simulink model "Sim_unicycle"  (R2024a)
settings: Solver=ode4  StartTime=0.0  StopTime=18  FixedStep=sample_time_continous  RelTol=1e-3
values from neighbouring files (symbols this model uses):
  sample_time_controller_outer = 1/10    (= 0.1)    [Main_quadrotor.m]    (also in Main_unicycle.m)
  sample_time_pathFG = sample_time_controller_outer    (= 0.1)    [Main_quadrotor.m]    (also in Main_unicycle.m)
  start = [0.1; 0.1; 0.3]    [Main_quadrotor.m]
undefined symbols (not defined in the file or in its folder): init_ref, init_state
settings Model: Creator=NewCrest Consulting  LastModifiedBy=serena
settings RTWCC: GPUComputeCapability=3.5

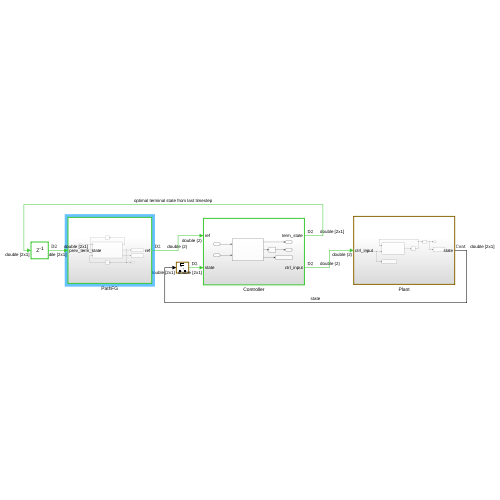
[thumbnail: Simulink's stored preview of the top-level diagram]
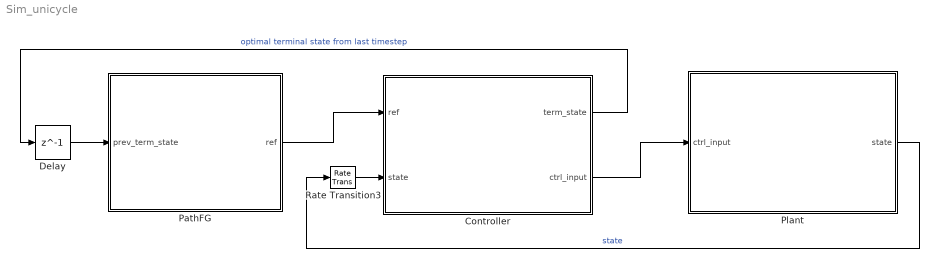
== system Sim_unicycle ==
  Controller : Subsystem
  Delay : Delay  DelayLength=1  InitialCondition=init_state
  PathFG : Subsystem  VariantControl=ref_source == 3
  Plant : Subsystem
  Rate Transition3 : RateTransition  InitialCondition=[start]  OutPortSampleTime=controller_sampling_time
  wires:
  Rate Transition3/1 -> Controller/2(state)
  Plant/1(state) -> Rate Transition3/1  "state"
  Delay/1 -> PathFG/1(prev_term_state)
  PathFG/1(ref) -> Controller/1(ref)
  Controller/1(term_state) -> Delay/1  "optimal terminal state from last timestep"
  Controller/2(ctrl_input) -> Plant/1(ctrl_input)

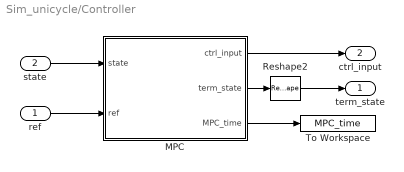
== system Sim_unicycle/Controller ==
  ref : Inport
  state : Inport  Port=2
  MPC : MATLAB Function  TreatAsAtomicUnit=on  SystemSampleTime=sample_time_controller_outer
  Reshape2 : Reshape  OutputDimensionality=Column vector (2-D)
  To Workspace : ToWorkspace  VariableName=MPC_time  SaveFormat=Timeseries  SampleTime=-1
  term_state : Outport
  ctrl_input : Outport  Port=2
  wires:
  ref/1 -> MPC/2(ref)
  state/1 -> MPC/1(state)
  MPC/3(MPC_time) -> To Workspace/1
  MPC/2(term_state) -> Reshape2/1
  MPC/1(ctrl_input) -> ctrl_input/1
  Reshape2/1 -> term_state/1

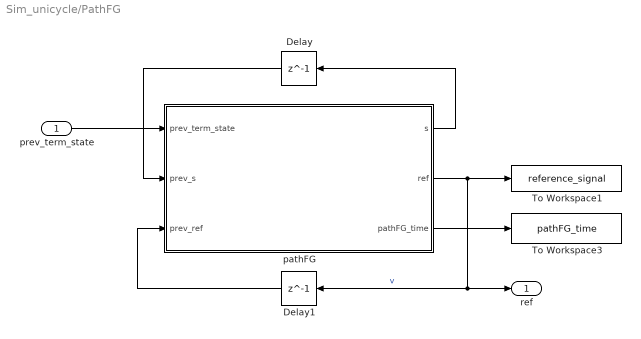
== system Sim_unicycle/PathFG ==
  prev_term_state : Inport
  Delay : Delay  DelayLength=1  InitialCondition=1
  Delay1 : Delay  DelayLength=1  InitialCondition=init_ref
  To Workspace1 : ToWorkspace  VariableName=reference_signal  SaveFormat=Timeseries  SampleTime=-1
  To Workspace3 : ToWorkspace  VariableName=pathFG_time  SaveFormat=Timeseries  SampleTime=-1
  pathFG : MATLAB Function  TreatAsAtomicUnit=on  SystemSampleTime=sample_time_pathFG
  ref : Outport
  wires:
  pathFG/2(ref) -> Delay1/1, ref/1, To Workspace1/1  "v"
  prev_term_state/1 -> pathFG/1(prev_term_state)
  pathFG/1(s) -> Delay/1
  Delay/1 -> pathFG/2(prev_s)
  Delay1/1 -> pathFG/3(prev_ref)
  pathFG/3(pathFG_time) -> To Workspace3/1

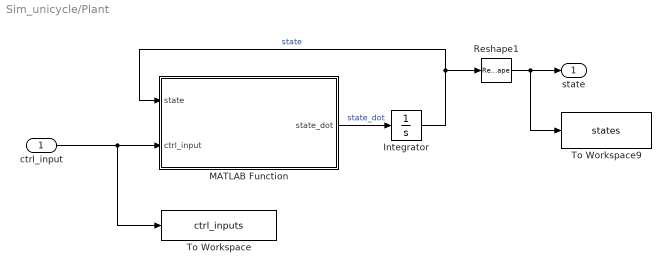
== system Sim_unicycle/Plant ==
  ctrl_input : Inport
  Integrator : Integrator  InitialCondition=init_state
  MATLAB Function : MATLAB Function  TreatAsAtomicUnit=on
  Reshape1 : Reshape  OutputDimensionality=Column vector (2-D)
  To Workspace : ToWorkspace  VariableName=ctrl_inputs  SaveFormat=Timeseries  SampleTime=-1
  To Workspace9 : ToWorkspace  VariableName=states  SaveFormat=Timeseries  SampleTime=-1
  state : Outport
  wires:
  Reshape1/1 -> state/1, To Workspace9/1
  Integrator/1 -> MATLAB Function/1(state), Reshape1/1  "state"
  MATLAB Function/1(state_dot) -> Integrator/1  "state_dot"
  ctrl_input/1 -> To Workspace/1, MATLAB Function/2(ctrl_input)

== matlab function Sim_unicycle/PathFG/pathFG ==
  settings: sampleTime=0.001
  data: s output; ref output; pathFG_time output; prev_term_state input; prev_s input; prev_ref input; params parameter
function [s, ref, pathFG_time] = callPathFG(prev_term_state, prev_s, prev_ref, params)

    N = params.N;
    pathFG_max_N = params.pathFG_max_N;
    path = params.path;
    path_size = params.path_size;

    pathFG_start = tic;
    if (N >= pathFG_max_N)
        s = path_size;
        ref = path(end,:)';  
        ref = reshape(ref, [], 1);
    else
        [s, ref] = pathFG(prev_term_state, prev_s, prev_ref, params);           
    end
    pathFG_time = toc(pathFG_start);
end

== matlab function Sim_unicycle/Controller/MPC ==
  data: ctrl_input output size=2; term_state output size=2; MPC_time output; state input; ref input; params parameter

function [ctrl_input, term_state, MPC_time] = callMPC(state, ref, params)
    % this allows fmincon to use the interior-point algorithm
    coder.extrinsic('MPC');
    MPC_start = tic;
    ctrl_input = zeros(2, 1);
    term_state = zeros(2, 1);
    [ctrl_input, term_state] = MPC(state, ref, params);
    MPC_time = toc(MPC_start);
end

== matlab function Sim_unicycle/Plant/MATLAB Function ==
  data: state input; state_dot output; ctrl_input input
% continuous time system equations
function state_dot = callContinuousEqs(state, ctrl_input)
    state_dot = unicycleContinuous(state, ctrl_input);
end
